simulink model "Multi_drones_deri_compare"  (R2021a)
settings: Solver=ode4  StartTime=0.0  StopTime=50  FixedStep=0.005  RelTol=1e-3
(part 1 of 7)
settings Model: Creator=a1752760  LastModifiedBy=a1752760

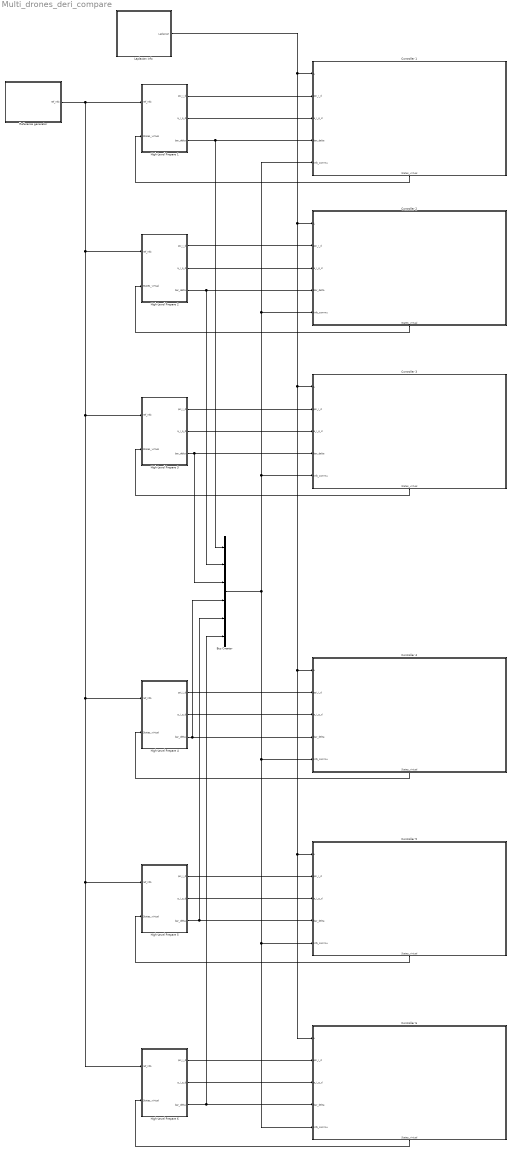
== system Multi_drones_deri_compare ==
  Bus Creator : BusCreator  Inputs=6
  Controller 1 : Subsystem
      settings: PortSchema="{\"entries\":[{\"content\":{\"sides\":[{\"content\":{\"connectorIds\":[\"In1\",\"In2\",\"In3\",\"In4\",\"In5\"]},\"type\":\"ConnectorPlacement.EquallySpacedRectSide\",\"uuid\":\"ede5c89e-e264-48e6-8668-eed849251501\"},{\"content\":{\"connectorIds\":[],\"side\":\"RIGHT\"},\"type\":\"ConnectorPlacement.EquallySpacedRectSide\",\"uuid\":\"e59691b4-d4b1-4407-a122-67eb4d4499aa\"},{\"content\":{\"connectorIds\":[],\"side\":\"TOP\"},\"type\":\"ConnectorPlacement.EquallySpacedRectSide\",\"uuid\":\"d9d52c18-65cc-4475-a64d-d3d1636b66e0\"},{\"content\":{\"connectorIds\":[\"Out1\"],\"side\":\"BOTTOM\"},\"type\":\"ConnectorPlacement.EquallySpacedRectSide\",\"uuid\":\"18635b8e-8039-4d54-8f78-9d501119f344\"}]},\"type\":\"ConnectorPlacement.EquallySpacedConnector\",\"uuid\":\"3cce6101-21cc-4dc7-9787-a7397180656f\"}],\"packageUris\":[\"http://schema.mathworks.com/mf0/Connector/R2020b\"],\"version\":\"1.0\"}"
  Controller 2 : Subsystem
      settings: PortSchema="{\"entries\":[{\"content\":{\"sides\":[{\"content\":{\"connectorIds\":[\"In1\",\"In2\",\"In3\",\"In4\",\"In5\"]},\"type\":\"ConnectorPlacement.EquallySpacedRectSide\",\"uuid\":\"ede5c89e-e264-48e6-8668-eed849251501\"},{\"content\":{\"connectorIds\":[],\"side\":\"RIGHT\"},\"type\":\"ConnectorPlacement.EquallySpacedRectSide\",\"uuid\":\"e59691b4-d4b1-4407-a122-67eb4d4499aa\"},{\"content\":{\"connectorIds\":[],\"side\":\"TOP\"},\"type\":\"ConnectorPlacement.EquallySpacedRectSide\",\"uuid\":\"d9d52c18-65cc-4475-a64d-d3d1636b66e0\"},{\"content\":{\"connectorIds\":[\"Out1\"],\"side\":\"BOTTOM\"},\"type\":\"ConnectorPlacement.EquallySpacedRectSide\",\"uuid\":\"18635b8e-8039-4d54-8f78-9d501119f344\"}]},\"type\":\"ConnectorPlacement.EquallySpacedConnector\",\"uuid\":\"3cce6101-21cc-4dc7-9787-a7397180656f\"}],\"packageUris\":[\"http://schema.mathworks.com/mf0/Connector/R2020b\"],\"version\":\"1.0\"}"
  Controller 3 : Subsystem
      settings: PortSchema="{\"entries\":[{\"content\":{\"sides\":[{\"content\":{\"connectorIds\":[\"In1\",\"In2\",\"In3\",\"In4\",\"In5\"]},\"type\":\"ConnectorPlacement.EquallySpacedRectSide\",\"uuid\":\"ede5c89e-e264-48e6-8668-eed849251501\"},{\"content\":{\"connectorIds\":[],\"side\":\"RIGHT\"},\"type\":\"ConnectorPlacement.EquallySpacedRectSide\",\"uuid\":\"e59691b4-d4b1-4407-a122-67eb4d4499aa\"},{\"content\":{\"connectorIds\":[],\"side\":\"TOP\"},\"type\":\"ConnectorPlacement.EquallySpacedRectSide\",\"uuid\":\"d9d52c18-65cc-4475-a64d-d3d1636b66e0\"},{\"content\":{\"connectorIds\":[\"Out1\"],\"side\":\"BOTTOM\"},\"type\":\"ConnectorPlacement.EquallySpacedRectSide\",\"uuid\":\"18635b8e-8039-4d54-8f78-9d501119f344\"}]},\"type\":\"ConnectorPlacement.EquallySpacedConnector\",\"uuid\":\"3cce6101-21cc-4dc7-9787-a7397180656f\"}],\"packageUris\":[\"http://schema.mathworks.com/mf0/Connector/R2020b\"],\"version\":\"1.0\"}"
  Controller 4 : Subsystem
      settings: PortSchema="{\"entries\":[{\"content\":{\"sides\":[{\"content\":{\"connectorIds\":[\"In1\",\"In2\",\"In3\",\"In4\",\"In5\"]},\"type\":\"ConnectorPlacement.EquallySpacedRectSide\",\"uuid\":\"ede5c89e-e264-48e6-8668-eed849251501\"},{\"content\":{\"connectorIds\":[],\"side\":\"RIGHT\"},\"type\":\"ConnectorPlacement.EquallySpacedRectSide\",\"uuid\":\"e59691b4-d4b1-4407-a122-67eb4d4499aa\"},{\"content\":{\"connectorIds\":[],\"side\":\"TOP\"},\"type\":\"ConnectorPlacement.EquallySpacedRectSide\",\"uuid\":\"d9d52c18-65cc-4475-a64d-d3d1636b66e0\"},{\"content\":{\"connectorIds\":[\"Out1\"],\"side\":\"BOTTOM\"},\"type\":\"ConnectorPlacement.EquallySpacedRectSide\",\"uuid\":\"18635b8e-8039-4d54-8f78-9d501119f344\"}]},\"type\":\"ConnectorPlacement.EquallySpacedConnector\",\"uuid\":\"3cce6101-21cc-4dc7-9787-a7397180656f\"}],\"packageUris\":[\"http://schema.mathworks.com/mf0/Connector/R2020b\"],\"version\":\"1.0\"}"
  Controller 5 : Subsystem
      settings: PortSchema="{\"entries\":[{\"content\":{\"sides\":[{\"content\":{\"connectorIds\":[\"In1\",\"In2\",\"In3\",\"In4\",\"In5\"]},\"type\":\"ConnectorPlacement.EquallySpacedRectSide\",\"uuid\":\"ede5c89e-e264-48e6-8668-eed849251501\"},{\"content\":{\"connectorIds\":[],\"side\":\"RIGHT\"},\"type\":\"ConnectorPlacement.EquallySpacedRectSide\",\"uuid\":\"e59691b4-d4b1-4407-a122-67eb4d4499aa\"},{\"content\":{\"connectorIds\":[],\"side\":\"TOP\"},\"type\":\"ConnectorPlacement.EquallySpacedRectSide\",\"uuid\":\"d9d52c18-65cc-4475-a64d-d3d1636b66e0\"},{\"content\":{\"connectorIds\":[\"Out1\"],\"side\":\"BOTTOM\"},\"type\":\"ConnectorPlacement.EquallySpacedRectSide\",\"uuid\":\"18635b8e-8039-4d54-8f78-9d501119f344\"}]},\"type\":\"ConnectorPlacement.EquallySpacedConnector\",\"uuid\":\"3cce6101-21cc-4dc7-9787-a7397180656f\"}],\"packageUris\":[\"http://schema.mathworks.com/mf0/Connector/R2020b\"],\"version\":\"1.0\"}"
  Controller 6 : Subsystem
      settings: PortSchema="{\"entries\":[{\"content\":{\"sides\":[{\"content\":{\"connectorIds\":[\"In1\",\"In2\",\"In3\",\"In4\",\"In5\"]},\"type\":\"ConnectorPlacement.EquallySpacedRectSide\",\"uuid\":\"ede5c89e-e264-48e6-8668-eed849251501\"},{\"content\":{\"connectorIds\":[],\"side\":\"RIGHT\"},\"type\":\"ConnectorPlacement.EquallySpacedRectSide\",\"uuid\":\"e59691b4-d4b1-4407-a122-67eb4d4499aa\"},{\"content\":{\"connectorIds\":[],\"side\":\"TOP\"},\"type\":\"ConnectorPlacement.EquallySpacedRectSide\",\"uuid\":\"d9d52c18-65cc-4475-a64d-d3d1636b66e0\"},{\"content\":{\"connectorIds\":[\"Out1\"],\"side\":\"BOTTOM\"},\"type\":\"ConnectorPlacement.EquallySpacedRectSide\",\"uuid\":\"18635b8e-8039-4d54-8f78-9d501119f344\"}]},\"type\":\"ConnectorPlacement.EquallySpacedConnector\",\"uuid\":\"3cce6101-21cc-4dc7-9787-a7397180656f\"}],\"packageUris\":[\"http://schema.mathworks.com/mf0/Connector/R2020b\"],\"version\":\"1.0\"}"
  High-Level Prepare 1 : Subsystem
  High-Level Prepare 2 : Subsystem
  High-Level Prepare 3 : Subsystem
  High-Level Prepare 4 : Subsystem
  High-Level Prepare 5 : Subsystem
  High-Level Prepare 6 : Subsystem
  Laplacian info : Subsystem
  Reference generator : Subsystem
  wires:
  Reference generator/1(ref_info) -> High-Level Prepare 6/1(ref_info), High-Level Prepare 5/1(ref_info), High-Level Prepare 4/1(ref_info), High-Level Prepare 3/1(ref_info), High-Level Prepare 2/1(ref_info), High-Level Prepare 1/1(ref_info)
  High-Level Prepare 1/1(psi_i_d) -> Controller 1/2(psi_i_d)
  High-Level Prepare 1/2(a_i_p_d) -> Controller 1/3(a_i_p_d)
  High-Level Prepare 1/3(bar_delta) -> Bus Creator/1, Controller 1/4(bar_delta)
  Controller 1/1(States_virtual) -> High-Level Prepare 1/2(States_virtual)
  Laplacian info/1(Laplacian) -> Controller 6/1(L), Controller 5/1(L), Controller 4/1(L), Controller 3/1(L), Controller 2/1(L), Controller 1/1(L)
  High-Level Prepare 2/2(a_i_p_d) -> Controller 2/3(a_i_p_d)
  High-Level Prepare 2/1(psi_i_d) -> Controller 2/2(psi_i_d)
  High-Level Prepare 2/3(bar_delta) -> Bus Creator/2, Controller 2/4(bar_delta)
  Controller 2/1(States_virtual) -> High-Level Prepare 2/2(States_virtual)
  High-Level Prepare 3/1(psi_i_d) -> Controller 3/2(psi_i_d)
  High-Level Prepare 3/3(bar_delta) -> Bus Creator/3, Controller 3/4(bar_delta)
  High-Level Prepare 3/2(a_i_p_d) -> Controller 3/3(a_i_p_d)
  Controller 3/1(States_virtual) -> High-Level Prepare 3/2(States_virtual)
  High-Level Prepare 4/1(psi_i_d) -> Controller 4/2(psi_i_d)
  High-Level Prepare 4/3(bar_delta) -> Bus Creator/4, Controller 4/4(bar_delta)
  High-Level Prepare 4/2(a_i_p_d) -> Controller 4/3(a_i_p_d)
  Controller 4/1(States_virtual) -> High-Level Prepare 4/2(States_virtual)
  High-Level Prepare 5/1(psi_i_d) -> Controller 5/2(psi_i_d)
  High-Level Prepare 5/3(bar_delta) -> Bus Creator/5, Controller 5/4(bar_delta)
  High-Level Prepare 5/2(a_i_p_d) -> Controller 5/3(a_i_p_d)
  Controller 5/1(States_virtual) -> High-Level Prepare 5/2(States_virtual)
  High-Level Prepare 6/1(psi_i_d) -> Controller 6/2(psi_i_d)
  High-Level Prepare 6/3(bar_delta) -> Bus Creator/6, Controller 6/4(bar_delta)
  High-Level Prepare 6/2(a_i_p_d) -> Controller 6/3(a_i_p_d)
  Controller 6/1(States_virtual) -> High-Level Prepare 6/2(States_virtual)
  Bus Creator/1 -> Controller 6/5(info_commu), Controller 5/5(info_commu), Controller 4/5(info_commu), Controller 2/5(info_commu), Controller 1/5(info_commu), Controller 3/5(info_commu)

== system Multi_drones_deri_compare/Controller 1 ==
  note: Change serial number and initial status
  note: Change serial number and initial status
  L : Inport
  psi_i_d : Inport  Port=2
  a_i_p_d : Inport  Port=3
  bar_delta : Inport  Port=4
  info_commu : Inport  Port=5
  Controller : Subsystem
  High-level system : Subsystem  mask{InitialCondition=[4;1;0]}
      mask prompts: InitialCondition "Simulink:blkprm_prompts:IntegratorInitCond"
      mask TypeOptions InitialCondition: bar_x/InitialCondition
      mask DialogControl InitialCondition Prompt: Initial condition:
  Quadcopter model : Subsystem  mask{InitialCondition=[4;1;0;0;0;0]}
      mask prompts: InitialCondition "Simulink:blkprm_prompts:IntegratorInitCond"
      mask TypeOptions InitialCondition: x_int/InitialCondition
      mask DialogControl InitialCondition Prompt: Initial condition:
  States_virtual : Outport
  wires:
  info_commu/1 -> High-level system/2(info_commu)
  bar_delta/1 -> High-level system/3(bar_delta)
  L/1 -> High-level system/1(L)
  a_i_p_d/1 -> High-level system/4(a_d)
  High-level system/2(States_virtual) -> States_virtual/1
  Controller/2(w_hat_p) -> Quadcopter model/2(w_hat_p)
  Quadcopter model/1(states_i) -> Controller/1(states_i)
  Controller/1(u_i) -> Quadcopter model/1(u_i)
  Controller/3(w_hat_a) -> Quadcopter model/3(w_hat_a)
  psi_i_d/1 -> Controller/3(psi_id)
  High-level system/1(new_ref) -> Controller/2(ref_x_p)

== system Multi_drones_deri_compare/Controller 2 ==
  note: Change serial number and initial status
  note: Change serial number and initial status
  L : Inport
  psi_i_d : Inport  Port=2
  a_i_p_d : Inport  Port=3
  bar_delta : Inport  Port=4
  info_commu : Inport  Port=5
  Controller : Subsystem
  High-level system : Subsystem  mask{InitialCondition=[1;2;0]}
      mask prompts: InitialCondition "Simulink:blkprm_prompts:IntegratorInitCond"
      mask TypeOptions InitialCondition: bar_x/InitialCondition
      mask DialogControl InitialCondition Prompt: Initial condition:
  Quadcopter model : Subsystem  mask{InitialCondition=[1;2;0;0;0;0]}
      mask prompts: InitialCondition "Simulink:blkprm_prompts:IntegratorInitCond"
      mask TypeOptions InitialCondition: x_int/InitialCondition
      mask DialogControl InitialCondition Prompt: Initial condition:
  States_virtual : Outport
  wires:
  info_commu/1 -> High-level system/2(info_commu)
  bar_delta/1 -> High-level system/3(bar_delta)
  L/1 -> High-level system/1(L)
  a_i_p_d/1 -> High-level system/4(a_d)
  High-level system/2(States_virtual) -> States_virtual/1
  Controller/2(w_hat_p) -> Quadcopter model/2(w_hat_p)
  Quadcopter model/1(states_i) -> Controller/1(states_i)
  Controller/1(u_i) -> Quadcopter model/1(u_i)
  Controller/3(w_hat_a) -> Quadcopter model/3(w_hat_a)
  psi_i_d/1 -> Controller/3(psi_id)
  High-level system/1(new_ref) -> Controller/2(ref_x_p)

== system Multi_drones_deri_compare/Controller 3 ==
  note: Change serial number and initial status
  note: Change serial number and initial status
  L : Inport
  psi_i_d : Inport  Port=2
  a_i_p_d : Inport  Port=3
  bar_delta : Inport  Port=4
  info_commu : Inport  Port=5
  Controller : Subsystem
  High-level system : Subsystem  mask{InitialCondition=[-2;4;0]}
      mask prompts: InitialCondition "Simulink:blkprm_prompts:IntegratorInitCond"
      mask TypeOptions InitialCondition: bar_x/InitialCondition
      mask DialogControl InitialCondition Prompt: Initial condition:
  Quadcopter model : Subsystem  mask{InitialCondition=[-2;4;0;0;0;0]}
      mask prompts: InitialCondition "Simulink:blkprm_prompts:IntegratorInitCond"
      mask TypeOptions InitialCondition: x_int/InitialCondition
      mask DialogControl InitialCondition Prompt: Initial condition:
  States_virtual : Outport
  wires:
  info_commu/1 -> High-level system/2(info_commu)
  bar_delta/1 -> High-level system/3(bar_delta)
  L/1 -> High-level system/1(L)
  a_i_p_d/1 -> High-level system/4(a_d)
  High-level system/2(States_virtual) -> States_virtual/1
  Controller/2(w_hat_p) -> Quadcopter model/2(w_hat_p)
  Quadcopter model/1(states_i) -> Controller/1(states_i)
  Controller/1(u_i) -> Quadcopter model/1(u_i)
  Controller/3(w_hat_a) -> Quadcopter model/3(w_hat_a)
  psi_i_d/1 -> Controller/3(psi_id)
  High-level system/1(new_ref) -> Controller/2(ref_x_p)

== system Multi_drones_deri_compare/Controller 4 ==
  note: Change serial number and initial status
  note: Change serial number and initial status
  L : Inport
  psi_i_d : Inport  Port=2
  a_i_p_d : Inport  Port=3
  bar_delta : Inport  Port=4
  info_commu : Inport  Port=5
  Controller : Subsystem
  High-level system : Subsystem  mask{InitialCondition=[-4;-1;0]}
      mask prompts: InitialCondition "Simulink:blkprm_prompts:IntegratorInitCond"
      mask TypeOptions InitialCondition: bar_x/InitialCondition
      mask DialogControl InitialCondition Prompt: Initial condition:
  Quadcopter model : Subsystem  mask{InitialCondition=[-4;-1;0;0;0;0]}
      mask prompts: InitialCondition "Simulink:blkprm_prompts:IntegratorInitCond"
      mask TypeOptions InitialCondition: x_int/InitialCondition
      mask DialogControl InitialCondition Prompt: Initial condition:
  States_virtual : Outport
  wires:
  info_commu/1 -> High-level system/2(info_commu)
  bar_delta/1 -> High-level system/3(bar_delta)
  L/1 -> High-level system/1(L)
  a_i_p_d/1 -> High-level system/4(a_d)
  High-level system/2(States_virtual) -> States_virtual/1
  Controller/2(w_hat_p) -> Quadcopter model/2(w_hat_p)
  Quadcopter model/1(states_i) -> Controller/1(states_i)
  Controller/1(u_i) -> Quadcopter model/1(u_i)
  Controller/3(w_hat_a) -> Quadcopter model/3(w_hat_a)
  psi_i_d/1 -> Controller/3(psi_id)
  High-level system/1(new_ref) -> Controller/2(ref_x_p)

== system Multi_drones_deri_compare/Controller 5 ==
  note: Change serial number and initial status
  note: Change serial number and initial status
  L : Inport
  psi_i_d : Inport  Port=2
  a_i_p_d : Inport  Port=3
  bar_delta : Inport  Port=4
  info_commu : Inport  Port=5
  Controller : Subsystem
  High-level system : Subsystem  mask{InitialCondition=[-1.5;-1;0]}
      mask prompts: InitialCondition "Simulink:blkprm_prompts:IntegratorInitCond"
      mask TypeOptions InitialCondition: bar_x/InitialCondition
      mask DialogControl InitialCondition Prompt: Initial condition:
  Quadcopter model : Subsystem  mask{InitialCondition=[-1.5;-1;0;0;0;0]}
      mask prompts: InitialCondition "Simulink:blkprm_prompts:IntegratorInitCond"
      mask TypeOptions InitialCondition: x_int/InitialCondition
      mask DialogControl InitialCondition Prompt: Initial condition:
  States_virtual : Outport
  wires:
  info_commu/1 -> High-level system/2(info_commu)
  bar_delta/1 -> High-level system/3(bar_delta)
  L/1 -> High-level system/1(L)
  a_i_p_d/1 -> High-level system/4(a_d)
  High-level system/2(States_virtual) -> States_virtual/1
  Controller/2(w_hat_p) -> Quadcopter model/2(w_hat_p)
  Quadcopter model/1(states_i) -> Controller/1(states_i)
  Controller/1(u_i) -> Quadcopter model/1(u_i)
  Controller/3(w_hat_a) -> Quadcopter model/3(w_hat_a)
  psi_i_d/1 -> Controller/3(psi_id)
  High-level system/1(new_ref) -> Controller/2(ref_x_p)

== system Multi_drones_deri_compare/Controller 6 ==
  note: Change serial number and initial status
  note: Change serial number and initial status
  L : Inport
  psi_i_d : Inport  Port=2
  a_i_p_d : Inport  Port=3
  bar_delta : Inport  Port=4
  info_commu : Inport  Port=5
  Controller : Subsystem
  High-level system : Subsystem  mask{InitialCondition=[0;-1;0]}
      mask prompts: InitialCondition "Simulink:blkprm_prompts:IntegratorInitCond"
      mask TypeOptions InitialCondition: bar_x/InitialCondition
      mask DialogControl InitialCondition Prompt: Initial condition:
  Quadcopter model : Subsystem  mask{InitialCondition=[0;-1;0;0;0;0]}
      mask prompts: InitialCondition "Simulink:blkprm_prompts:IntegratorInitCond"
      mask TypeOptions InitialCondition: x_int/InitialCondition
      mask DialogControl InitialCondition Prompt: Initial condition:
  States_virtual : Outport
  wires:
  info_commu/1 -> High-level system/2(info_commu)
  bar_delta/1 -> High-level system/3(bar_delta)
  L/1 -> High-level system/1(L)
  a_i_p_d/1 -> High-level system/4(a_d)
  High-level system/2(States_virtual) -> States_virtual/1
  Controller/2(w_hat_p) -> Quadcopter model/2(w_hat_p)
  Quadcopter model/1(states_i) -> Controller/1(states_i)
  Controller/1(u_i) -> Quadcopter model/1(u_i)
  Controller/3(w_hat_a) -> Quadcopter model/3(w_hat_a)
  psi_i_d/1 -> Controller/3(psi_id)
  High-level system/1(new_ref) -> Controller/2(ref_x_p)

== system Multi_drones_deri_compare/High-Level Prepare 1 ==
  note: Change serial number here
  ref_info : Inport
  States_virtual : Inport  Port=2
  Bus Creator : BusCreator  Inputs=2
  Reference selection (Low) : MATLAB Function  TreatAsAtomicUnit=on
  States selection (Virtual) : MATLAB Function  TreatAsAtomicUnit=on
  Virtual error calculation : MATLAB Function  TreatAsAtomicUnit=on
  psi_i_d : Outport
  a_i_p_d : Outport  Port=2
  bar_delta : Outport  Port=3
  wires:
  ref_info/1 -> Reference selection (Low)/1(ref_info)
  Reference selection (Low)/4(psi_i_d) -> psi_i_d/1
  States_virtual/1 -> States selection (Virtual)/1(states_virtual)
  Reference selection (Low)/3(a_i_p_d) -> a_i_p_d/1
  States selection (Virtual)/2(v_bar_i) -> Virtual error calculation/2(v_bar_i)
  States selection (Virtual)/1(x_bar_i) -> Virtual error calculation/1(x_bar_i)
  Reference selection (Low)/1(x_i_p_d) -> Virtual error calculation/3(x_i_p_d)
  Reference selection (Low)/2(v_i_p_d) -> Virtual error calculation/4(v_i_p_d)
  Virtual error calculation/1(bar_delta_x) -> Bus Creator/1
  Virtual error calculation/2(bar_delta_v) -> Bus Creator/2
  Bus Creator/1 -> bar_delta/1

== system Multi_drones_deri_compare/High-Level Prepare 2 ==
  note: Change serial number here
  ref_info : Inport
  States_virtual : Inport  Port=2
  Bus Creator : BusCreator  Inputs=2
  Reference selection (Low) : MATLAB Function  TreatAsAtomicUnit=on
  States selection (Virtual) : MATLAB Function  TreatAsAtomicUnit=on
  Virtual error calculation : MATLAB Function  TreatAsAtomicUnit=on
  psi_i_d : Outport
  a_i_p_d : Outport  Port=2
  bar_delta : Outport  Port=3
  wires:
  ref_info/1 -> Reference selection (Low)/1(ref_info)
  Reference selection (Low)/4(psi_i_d) -> psi_i_d/1
  States_virtual/1 -> States selection (Virtual)/1(states_virtual)
  Reference selection (Low)/3(a_i_p_d) -> a_i_p_d/1
  States selection (Virtual)/2(v_bar_i) -> Virtual error calculation/2(v_bar_i)
  States selection (Virtual)/1(x_bar_i) -> Virtual error calculation/1(x_bar_i)
  Reference selection (Low)/1(x_i_p_d) -> Virtual error calculation/3(x_i_p_d)
  Reference selection (Low)/2(v_i_p_d) -> Virtual error calculation/4(v_i_p_d)
  Virtual error calculation/1(bar_delta_x) -> Bus Creator/1
  Virtual error calculation/2(bar_delta_v) -> Bus Creator/2
  Bus Creator/1 -> bar_delta/1

== system Multi_drones_deri_compare/High-Level Prepare 3 ==
  note: Change serial number here
  ref_info : Inport
  States_virtual : Inport  Port=2
  Bus Creator : BusCreator  Inputs=2
  Reference selection (Low) : MATLAB Function  TreatAsAtomicUnit=on
  States selection (Virtual) : MATLAB Function  TreatAsAtomicUnit=on
  Virtual error calculation : MATLAB Function  TreatAsAtomicUnit=on
  psi_i_d : Outport
  a_i_p_d : Outport  Port=2
  bar_delta : Outport  Port=3
  wires:
  ref_info/1 -> Reference selection (Low)/1(ref_info)
  Reference selection (Low)/4(psi_i_d) -> psi_i_d/1
  States_virtual/1 -> States selection (Virtual)/1(states_virtual)
  Reference selection (Low)/3(a_i_p_d) -> a_i_p_d/1
  States selection (Virtual)/2(v_bar_i) -> Virtual error calculation/2(v_bar_i)
  States selection (Virtual)/1(x_bar_i) -> Virtual error calculation/1(x_bar_i)
  Reference selection (Low)/1(x_i_p_d) -> Virtual error calculation/3(x_i_p_d)
  Reference selection (Low)/2(v_i_p_d) -> Virtual error calculation/4(v_i_p_d)
  Virtual error calculation/1(bar_delta_x) -> Bus Creator/1
  Virtual error calculation/2(bar_delta_v) -> Bus Creator/2
  Bus Creator/1 -> bar_delta/1

== system Multi_drones_deri_compare/High-Level Prepare 4 ==
  note: Change serial number here
  ref_info : Inport
  States_virtual : Inport  Port=2
  Bus Creator : BusCreator  Inputs=2
  Reference selection (Low) : MATLAB Function  TreatAsAtomicUnit=on
  States selection (Virtual) : MATLAB Function  TreatAsAtomicUnit=on
  Virtual error calculation : MATLAB Function  TreatAsAtomicUnit=on
  psi_i_d : Outport
  a_i_p_d : Outport  Port=2
  bar_delta : Outport  Port=3
  wires:
  ref_info/1 -> Reference selection (Low)/1(ref_info)
  Reference selection (Low)/4(psi_i_d) -> psi_i_d/1
  States_virtual/1 -> States selection (Virtual)/1(states_virtual)
  Reference selection (Low)/3(a_i_p_d) -> a_i_p_d/1
  States selection (Virtual)/2(v_bar_i) -> Virtual error calculation/2(v_bar_i)
  States selection (Virtual)/1(x_bar_i) -> Virtual error calculation/1(x_bar_i)
  Reference selection (Low)/1(x_i_p_d) -> Virtual error calculation/3(x_i_p_d)
  Reference selection (Low)/2(v_i_p_d) -> Virtual error calculation/4(v_i_p_d)
  Virtual error calculation/1(bar_delta_x) -> Bus Creator/1
  Virtual error calculation/2(bar_delta_v) -> Bus Creator/2
  Bus Creator/1 -> bar_delta/1

== system Multi_drones_deri_compare/High-Level Prepare 5 ==
  note: Change serial number here
  ref_info : Inport
  States_virtual : Inport  Port=2
  Bus Creator : BusCreator  Inputs=2
  Reference selection (Low) : MATLAB Function  TreatAsAtomicUnit=on
  States selection (Virtual) : MATLAB Function  TreatAsAtomicUnit=on
  Virtual error calculation : MATLAB Function  TreatAsAtomicUnit=on
  psi_i_d : Outport
  a_i_p_d : Outport  Port=2
  bar_delta : Outport  Port=3
  wires:
  ref_info/1 -> Reference selection (Low)/1(ref_info)
  Reference selection (Low)/4(psi_i_d) -> psi_i_d/1
  States_virtual/1 -> States selection (Virtual)/1(states_virtual)
  Reference selection (Low)/3(a_i_p_d) -> a_i_p_d/1
  States selection (Virtual)/2(v_bar_i) -> Virtual error calculation/2(v_bar_i)
  States selection (Virtual)/1(x_bar_i) -> Virtual error calculation/1(x_bar_i)
  Reference selection (Low)/1(x_i_p_d) -> Virtual error calculation/3(x_i_p_d)
  Reference selection (Low)/2(v_i_p_d) -> Virtual error calculation/4(v_i_p_d)
  Virtual error calculation/1(bar_delta_x) -> Bus Creator/1
  Virtual error calculation/2(bar_delta_v) -> Bus Creator/2
  Bus Creator/1 -> bar_delta/1

== system Multi_drones_deri_compare/High-Level Prepare 6 ==
  note: Change serial number here
  ref_info : Inport
  States_virtual : Inport  Port=2
  Bus Creator : BusCreator  Inputs=2
  Reference selection (Low) : MATLAB Function  TreatAsAtomicUnit=on
  States selection (Virtual) : MATLAB Function  TreatAsAtomicUnit=on
  Virtual error calculation : MATLAB Function  TreatAsAtomicUnit=on
  psi_i_d : Outport
  a_i_p_d : Outport  Port=2
  bar_delta : Outport  Port=3
  wires:
  ref_info/1 -> Reference selection (Low)/1(ref_info)
  Reference selection (Low)/4(psi_i_d) -> psi_i_d/1
  States_virtual/1 -> States selection (Virtual)/1(states_virtual)
  Reference selection (Low)/3(a_i_p_d) -> a_i_p_d/1
  States selection (Virtual)/2(v_bar_i) -> Virtual error calculation/2(v_bar_i)
  States selection (Virtual)/1(x_bar_i) -> Virtual error calculation/1(x_bar_i)
  Reference selection (Low)/1(x_i_p_d) -> Virtual error calculation/3(x_i_p_d)
  Reference selection (Low)/2(v_i_p_d) -> Virtual error calculation/4(v_i_p_d)
  Virtual error calculation/1(bar_delta_x) -> Bus Creator/1
  Virtual error calculation/2(bar_delta_v) -> Bus Creator/2
  Bus Creator/1 -> bar_delta/1

== system Multi_drones_deri_compare/Laplacian info ==
  Add : Sum
  Communication topology : MATLAB Function  TreatAsAtomicUnit=on
  Constant : Constant  Value=diag(ones(6,1))  VectorParams1D=off
  Multiply : Gain
  Laplacian : Outport
  wires:
  Constant/1 -> Multiply/1
  Multiply/1 -> Add/1
  Add/1 -> Laplacian/1
  Communication topology/1(L) -> Add/2

== system Multi_drones_deri_compare/Reference generator ==
  Bus Creator : BusCreator  Inputs=4
  Coordinate reference : Subsystem
  MATLAB Function : MATLAB Function  TreatAsAtomicUnit=on
  Scope : Scope
  Simulation time : Clock
  ref_info : Outport
  wires:
  Simulation time/1 -> Coordinate reference/1(Time), MATLAB Function/1(t)
  Coordinate reference/1(x_d_p) -> Scope/1, Bus Creator/1
  Coordinate reference/2(v_d_p) -> Bus Creator/2
  Coordinate reference/3(a_d_p) -> Bus Creator/3
  MATLAB Function/1(x_d_a) -> Bus Creator/4
  Bus Creator/1 -> ref_info/1

== system Multi_drones_deri_compare/Controller 1/Controller ==
  note: Change the serial number here
  note: Change the serial number here
  note: Change the serial number here
  states_i : Inport
  ref_x_p : Inport  Port=2
  psi_id : Inport  Port=3
  Attitude controller : Subsystem
      settings: PortSchema="{\"entries\":[{\"content\":{\"sides\":[{\"content\":{\"connectorIds\":[\"In1\",\"In2\",\"In3\"]},\"type\":\"ConnectorPlacement.EquallySpacedRectSide\",\"uuid\":\"fa62b1eb-ed3d-4a84-b897-b51f17bb9d42\"},{\"content\":{\"connectorIds\":[\"Out1\"],\"side\":\"RIGHT\"},\"type\":\"ConnectorPlacement.EquallySpacedRectSide\",\"uuid\":\"9b6b7a3c-e484-45bf-bd32-fe40ffeb0d28\"},{\"content\":{\"connectorIds\":[\"Out2\"],\"side\":\"TOP\"},\"type\":\"ConnectorPlacement.EquallySpacedRectSide\",\"uuid\":\"d1ffdbb9-18c9-4f2c-95a6-bf4c2ab27347\"}]},\"type\":\"ConnectorPlacement.EquallySpacedConnector\",\"uuid\":\"2804a1df-60db-43d6-95d2-4687dde4bd06\"}],\"packageUris\":[\"http://schema.mathworks.com/mf0/Connector/R2020b\"],\"version\":\"1.0\"}"
  Constant : Constant  Value=13.72  VectorParams1D=off
  Manual Switch : ManualSwitch
  Nominal control calculation : MATLAB Function  TreatAsAtomicUnit=on
  Position controller1 : Subsystem
      settings: PortSchema="{\"entries\":[{\"content\":{\"sides\":[{\"content\":{\"connectorIds\":[\"In1\",\"In2\",\"In3\"]},\"type\":\"ConnectorPlacement.EquallySpacedRectSide\",\"uuid\":\"6f6db54a-065c-4c68-96d3-ce6f9528f7c2\"},{\"content\":{\"connectorIds\":[\"Out1\"],\"side\":\"RIGHT\"},\"type\":\"ConnectorPlacement.EquallySpacedRectSide\",\"uuid\":\"eab021de-0481-49e0-8239-dbc5993eb5fa\"},{\"content\":{\"connectorIds\":[\"Out2\"],\"side\":\"TOP\"},\"type\":\"ConnectorPlacement.EquallySpacedRectSide\",\"uuid\":\"c7d044cf-1b8b-40e5-8601-940ebebd0ccb\"},{\"content\":{\"connectorIds\":[],\"side\":\"BOTTOM\"},\"type\":\"ConnectorPlacement.EquallySpacedRectSide\",\"uuid\":\"6c5daa93-b438-4c34-9741-3ab1f6346320\"}]},\"type\":\"ConnectorPlacement.EquallySpacedConnector\",\"uuid\":\"bb7db914-9823-41d6-a8ba-39b4d2976335\"}],\"packageUris\":[\"http://schema.mathworks.com/mf0/Connector/R2020b\"],\"version\":\"1.0\"}"
  Real control input : MATLAB Function  TreatAsAtomicUnit=on
  Reverse calculation : Subsystem
      settings: PortSchema="{\"entries\":[{\"content\":{\"sides\":[{\"content\":{\"connectorIds\":[\"In1\",\"In2\"]},\"type\":\"ConnectorPlacement.EquallySpacedRectSide\",\"uuid\":\"a324fb00-881d-40c1-b7da-a9c7871d46ce\"},{\"content\":{\"connectorIds\":[\"Out1\",\"Out2\"],\"side\":\"RIGHT\"},\"type\":\"ConnectorPlacement.EquallySpacedRectSide\",\"uuid\":\"58739d0b-b2b3-44e8-8796-6553ce8d5a15\"},{\"content\":{\"connectorIds\":[\"In3\"],\"side\":\"TOP\"},\"type\":\"ConnectorPlacement.EquallySpacedRectSide\",\"uuid\":\"8c9acd48-a842-4889-b739-8799f04ac800\"}]},\"type\":\"ConnectorPlacement.EquallySpacedConnector\",\"uuid\":\"9c847f57-6425-42e5-8be7-b64809e08636\"}],\"packageUris\":[\"http://schema.mathworks.com/mf0/Connector/R2020b\"],\"version\":\"1.0\"}"
  Scope : Scope
  T_id : Scope
  atti_ref : Scope
  u : Scope
  u_ip : Scope
  u_nom_a : Scope
  u_nom_p : Scope
  u_i : Outport
  w_hat_p : Outport  Port=2
  w_hat_a : Outport  Port=3
  wires:
  Attitude controller/1(u_I_a) -> Real control input/1(u_i_a)
  ref_x_p/1 -> Position controller1/2(ref_x_p)
  states_i/1 -> Position controller1/1(states_i), Reverse calculation/3(states_i), Attitude controller/1(states_i), Nominal control calculation/1(states_i)
  Nominal control calculation/1(u_nom_p) -> Position controller1/3(u_nom_p), u_nom_p/1
  Nominal control calculation/2(u_nom_a) -> Attitude controller/3(u_nom_a), u_nom_a/1
  Position controller1/1(u_i_p) -> Reverse calculation/2(u_ip), u_ip/1
  Reverse calculation/1(atti_ref) -> Attitude controller/2(atti_ref), atti_ref/1
  Position controller1/2(w_hat_p) -> w_hat_p/1
  Attitude controller/2(w_hat_a) -> w_hat_a/1
  Constant/1 -> Manual Switch/2
  Reverse calculation/2(T_i_d) -> Manual Switch/1
  Manual Switch/1 -> T_id/1, Real control input/2(T_id)
  Real control input/2(u_i) -> Nominal control calculation/2(u_i), u/1, u_i/1
  Real control input/1(tau_i) -> Scope/1
  psi_id/1 -> Reverse calculation/1(psi_id)

== system Multi_drones_deri_compare/Controller 1/High-level system ==
  L : Inport
  info_commu : Inport  Port=2
  bar_delta : Inport  Port=3
  a_d : Inport  Port=4
  Bus Creator : BusCreator  Inputs=3
  Bus Creator1 : BusCreator  Inputs=2
  Controller : MATLAB Function  TreatAsAtomicUnit=on
  Information subtracting : MATLAB Function  TreatAsAtomicUnit=on
  Saturation : Saturate  UpperLimit=0.2  LowerLimit=-0.2
  Virtual sliding variable : Scope
  Virtual tracking error : Scope
  bar_u_i : Scope
  bar_v : Integrator  InitialCondition=[0;0;0]  ContinuousStateAttributes='speed'
  bar_v_i : Scope
  bar_x : Integrator  Tag=Position_x1  InitialCondition=InitialCondition  ContinuousStateAttributes='position'
  bar_x_i : Scope
  new_ref : Outport
  States_virtual : Outport  Port=2
  wires:
  Information subtracting/1(delta_xi) -> Controller/1(delta_xi), Virtual tracking error/1
  Information subtracting/2(delta_vi) -> Controller/2(delta_vi)
  Information subtracting/3(s_i) -> Virtual sliding variable/1, Controller/3(s_i)
  info_commu/1 -> Information subtracting/2(info_commu)
  bar_delta/1 -> Information subtracting/3(bar_delta)
  L/1 -> Information subtracting/1(L)
  a_d/1 -> Controller/5(a_di)
  bar_v/1 -> Bus Creator1/2, bar_v_i/1, Bus Creator/2, bar_x/1
  Bus Creator/1 -> new_ref/1
  bar_x/1 -> Bus Creator1/1, Bus Creator/1, bar_x_i/1
  Bus Creator1/1 -> States_virtual/1
  Controller/1(u_i) -> Saturation/1
  Saturation/1 -> bar_u_i/1, Bus Creator/3, bar_v/1
  Information subtracting/4(sat_dot) -> Controller/4(sat_dot)

== system Multi_drones_deri_compare/Controller 1/Quadcopter model ==
  u_i : Inport
  w_hat_p : Inport  Port=2
  w_hat_a : Inport  Port=3
  Add : Sum  Inputs=+-
  Add1 : Sum  Inputs=+-
  Bus Creator : BusCreator  Inputs=2
  Clock : Clock
  Quadcopter dynamics : MATLAB Function  TreatAsAtomicUnit=on
  f_a : Scope
  f_p : Scope
  quad_v : Scope
  quad_x : Scope
  v_int : Integrator  InitialCondition=[0;0;0;0;0;0]
  w_tilde_a : Scope
  w_tilde_p : Scope
  x_int : Integrator  InitialCondition=InitialCondition
  states_i : Outport
  wires:
  u_i/1 -> Quadcopter dynamics/2(u_i)
  Quadcopter dynamics/1(x_ddot) -> v_int/1
  x_int/1 -> Quadcopter dynamics/1(x_i), quad_x/1, Bus Creator/1
  v_int/1 -> Bus Creator/2, quad_v/1, Quadcopter dynamics/4(v_i), x_int/1
  Bus Creator/1 -> states_i/1
  Quadcopter dynamics/2(w_a) -> Add/1, f_a/1
  w_hat_a/1 -> Add/2
  Add/1 -> w_tilde_a/1
  Clock/1 -> Quadcopter dynamics/3(t)
  Quadcopter dynamics/3(w_p) -> f_p/1, Add1/1
  w_hat_p/1 -> Add1/2
  Add1/1 -> w_tilde_p/1

== system Multi_drones_deri_compare/Controller 2/Controller ==
  note: Change the serial number here
  note: Change the serial number here
  note: Change the serial number here
  states_i : Inport
  ref_x_p : Inport  Port=2
  psi_id : Inport  Port=3
  Attitude controller : Subsystem
      settings: PortSchema="{\"entries\":[{\"content\":{\"sides\":[{\"content\":{\"connectorIds\":[\"In1\",\"In2\",\"In3\"]},\"type\":\"ConnectorPlacement.EquallySpacedRectSide\",\"uuid\":\"fa62b1eb-ed3d-4a84-b897-b51f17bb9d42\"},{\"content\":{\"connectorIds\":[\"Out1\"],\"side\":\"RIGHT\"},\"type\":\"ConnectorPlacement.EquallySpacedRectSide\",\"uuid\":\"9b6b7a3c-e484-45bf-bd32-fe40ffeb0d28\"},{\"content\":{\"connectorIds\":[\"Out2\"],\"side\":\"TOP\"},\"type\":\"ConnectorPlacement.EquallySpacedRectSide\",\"uuid\":\"d1ffdbb9-18c9-4f2c-95a6-bf4c2ab27347\"}]},\"type\":\"ConnectorPlacement.EquallySpacedConnector\",\"uuid\":\"2804a1df-60db-43d6-95d2-4687dde4bd06\"}],\"packageUris\":[\"http://schema.mathworks.com/mf0/Connector/R2020b\"],\"version\":\"1.0\"}"
  Constant : Constant  Value=13.72  VectorParams1D=off
  Manual Switch : ManualSwitch
  Nominal control calculation : MATLAB Function  TreatAsAtomicUnit=on
  Position controller1 : Subsystem
      settings: PortSchema="{\"entries\":[{\"content\":{\"sides\":[{\"content\":{\"connectorIds\":[\"In1\",\"In2\",\"In3\"]},\"type\":\"ConnectorPlacement.EquallySpacedRectSide\",\"uuid\":\"6f6db54a-065c-4c68-96d3-ce6f9528f7c2\"},{\"content\":{\"connectorIds\":[\"Out1\"],\"side\":\"RIGHT\"},\"type\":\"ConnectorPlacement.EquallySpacedRectSide\",\"uuid\":\"eab021de-0481-49e0-8239-dbc5993eb5fa\"},{\"content\":{\"connectorIds\":[\"Out2\"],\"side\":\"TOP\"},\"type\":\"ConnectorPlacement.EquallySpacedRectSide\",\"uuid\":\"c7d044cf-1b8b-40e5-8601-940ebebd0ccb\"},{\"content\":{\"connectorIds\":[],\"side\":\"BOTTOM\"},\"type\":\"ConnectorPlacement.EquallySpacedRectSide\",\"uuid\":\"6c5daa93-b438-4c34-9741-3ab1f6346320\"}]},\"type\":\"ConnectorPlacement.EquallySpacedConnector\",\"uuid\":\"bb7db914-9823-41d6-a8ba-39b4d2976335\"}],\"packageUris\":[\"http://schema.mathworks.com/mf0/Connector/R2020b\"],\"version\":\"1.0\"}"
  Real control input : MATLAB Function  TreatAsAtomicUnit=on
  Reverse calculation : Subsystem
      settings: PortSchema="{\"entries\":[{\"content\":{\"sides\":[{\"content\":{\"connectorIds\":[\"In1\",\"In2\"]},\"type\":\"ConnectorPlacement.EquallySpacedRectSide\",\"uuid\":\"a324fb00-881d-40c1-b7da-a9c7871d46ce\"},{\"content\":{\"connectorIds\":[\"Out1\",\"Out2\"],\"side\":\"RIGHT\"},\"type\":\"ConnectorPlacement.EquallySpacedRectSide\",\"uuid\":\"58739d0b-b2b3-44e8-8796-6553ce8d5a15\"},{\"content\":{\"connectorIds\":[\"In3\"],\"side\":\"TOP\"},\"type\":\"ConnectorPlacement.EquallySpacedRectSide\",\"uuid\":\"8c9acd48-a842-4889-b739-8799f04ac800\"}]},\"type\":\"ConnectorPlacement.EquallySpacedConnector\",\"uuid\":\"9c847f57-6425-42e5-8be7-b64809e08636\"}],\"packageUris\":[\"http://schema.mathworks.com/mf0/Connector/R2020b\"],\"version\":\"1.0\"}"
  Scope : Scope
  T_id : Scope
  atti_ref : Scope
  u : Scope
  u_ip : Scope
  u_nom_a : Scope
  u_nom_p : Scope
  u_i : Outport
  w_hat_p : Outport  Port=2
  w_hat_a : Outport  Port=3
  wires:
  Attitude controller/1(u_I_a) -> Real control input/1(u_i_a)
  ref_x_p/1 -> Position controller1/2(ref_x_p)
  states_i/1 -> Position controller1/1(states_i), Reverse calculation/3(states_i), Attitude controller/1(states_i), Nominal control calculation/1(states_i)
  Nominal control calculation/1(u_nom_p) -> Position controller1/3(u_nom_p), u_nom_p/1
  Nominal control calculation/2(u_nom_a) -> Attitude controller/3(u_nom_a), u_nom_a/1
  Position controller1/1(u_i_p) -> Reverse calculation/2(u_ip), u_ip/1
  Reverse calculation/1(atti_ref) -> Attitude controller/2(atti_ref), atti_ref/1
  Position controller1/2(w_hat_p) -> w_hat_p/1
  Attitude controller/2(w_hat_a) -> w_hat_a/1
  Constant/1 -> Manual Switch/2
  Reverse calculation/2(T_i_d) -> Manual Switch/1
  Manual Switch/1 -> T_id/1, Real control input/2(T_id)
  Real control input/2(u_i) -> Nominal control calculation/2(u_i), u/1, u_i/1
  Real control input/1(tau_i) -> Scope/1
  psi_id/1 -> Reverse calculation/1(psi_id)

== system Multi_drones_deri_compare/Controller 2/High-level system ==
  L : Inport
  info_commu : Inport  Port=2
  bar_delta : Inport  Port=3
  a_d : Inport  Port=4
  Bus Creator : BusCreator  Inputs=3
  Bus Creator1 : BusCreator  Inputs=2
  Controller : MATLAB Function  TreatAsAtomicUnit=on
  Information subtracting : MATLAB Function  TreatAsAtomicUnit=on
  Saturation : Saturate  UpperLimit=0.2  LowerLimit=-0.2
  Virtual sliding variable : Scope
  Virtual tracking error : Scope
  bar_u_i : Scope
  bar_v : Integrator  InitialCondition=[0;0;0]  ContinuousStateAttributes='speed'
  bar_v_i : Scope
  bar_x : Integrator  Tag=Position_x1  InitialCondition=InitialCondition  ContinuousStateAttributes='position'
  bar_x_i : Scope
  new_ref : Outport
  States_virtual : Outport  Port=2
  wires:
  Information subtracting/1(delta_xi) -> Controller/1(delta_xi), Virtual tracking error/1
  Information subtracting/4(sat_dot) -> Controller/4(sat_dot)
  info_commu/1 -> Information subtracting/2(info_commu)
  bar_delta/1 -> Information subtracting/3(bar_delta)
  L/1 -> Information subtracting/1(L)
  a_d/1 -> Controller/5(a_di)
  bar_v/1 -> Bus Creator1/2, bar_v_i/1, Bus Creator/2, bar_x/1
  Bus Creator/1 -> new_ref/1
  bar_x/1 -> Bus Creator1/1, Bus Creator/1, bar_x_i/1
  Bus Creator1/1 -> States_virtual/1
  Controller/1(u_i) -> Saturation/1
  Saturation/1 -> bar_u_i/1, Bus Creator/3, bar_v/1
  Information subtracting/2(delta_vi) -> Controller/2(delta_vi)
  Information subtracting/3(s_i) -> Controller/3(s_i), Virtual sliding variable/1

== system Multi_drones_deri_compare/Controller 2/Quadcopter model ==
  u_i : Inport
  w_hat_p : Inport  Port=2
  w_hat_a : Inport  Port=3
  Add : Sum  Inputs=+-
  Add1 : Sum  Inputs=+-
  Bus Creator : BusCreator  Inputs=2
  Clock : Clock
  Quadcopter dynamics : MATLAB Function  TreatAsAtomicUnit=on
  f_a : Scope
  f_p : Scope
  quad_v : Scope
  quad_x : Scope
  v_int : Integrator  InitialCondition=[0;0;0;0;0;0]
  w_tilde_a_2 : Scope
  w_tilde_p_2 : Scope
  x_int : Integrator  InitialCondition=InitialCondition
  states_i : Outport
  wires:
  u_i/1 -> Quadcopter dynamics/2(u_i)
  Quadcopter dynamics/1(x_ddot) -> v_int/1
  x_int/1 -> Quadcopter dynamics/1(x_i), quad_x/1, Bus Creator/1
  v_int/1 -> Bus Creator/2, quad_v/1, Quadcopter dynamics/4(v_i), x_int/1
  Bus Creator/1 -> states_i/1
  Quadcopter dynamics/2(w_a) -> Add/1, f_a/1
  w_hat_a/1 -> Add/2
  Add/1 -> w_tilde_a_2/1
  Clock/1 -> Quadcopter dynamics/3(t)
  Quadcopter dynamics/3(w_p) -> f_p/1, Add1/1
  w_hat_p/1 -> Add1/2
  Add1/1 -> w_tilde_p_2/1

== system Multi_drones_deri_compare/Controller 3/Controller ==
  note: Change the serial number here
  note: Change the serial number here
  note: Change the serial number here
  states_i : Inport
  ref_x_p : Inport  Port=2
  psi_id : Inport  Port=3
  Attitude controller : Subsystem
      settings: PortSchema="{\"entries\":[{\"content\":{\"sides\":[{\"content\":{\"connectorIds\":[\"In1\",\"In2\",\"In3\"]},\"type\":\"ConnectorPlacement.EquallySpacedRectSide\",\"uuid\":\"fa62b1eb-ed3d-4a84-b897-b51f17bb9d42\"},{\"content\":{\"connectorIds\":[\"Out1\"],\"side\":\"RIGHT\"},\"type\":\"ConnectorPlacement.EquallySpacedRectSide\",\"uuid\":\"9b6b7a3c-e484-45bf-bd32-fe40ffeb0d28\"},{\"content\":{\"connectorIds\":[\"Out2\"],\"side\":\"TOP\"},\"type\":\"ConnectorPlacement.EquallySpacedRectSide\",\"uuid\":\"d1ffdbb9-18c9-4f2c-95a6-bf4c2ab27347\"}]},\"type\":\"ConnectorPlacement.EquallySpacedConnector\",\"uuid\":\"2804a1df-60db-43d6-95d2-4687dde4bd06\"}],\"packageUris\":[\"http://schema.mathworks.com/mf0/Connector/R2020b\"],\"version\":\"1.0\"}"
  Constant : Constant  Value=13.72  VectorParams1D=off
  Manual Switch : ManualSwitch
  Nominal control calculation : MATLAB Function  TreatAsAtomicUnit=on
  Position controller1 : Subsystem
      settings: PortSchema="{\"entries\":[{\"content\":{\"sides\":[{\"content\":{\"connectorIds\":[\"In1\",\"In2\",\"In3\"]},\"type\":\"ConnectorPlacement.EquallySpacedRectSide\",\"uuid\":\"6f6db54a-065c-4c68-96d3-ce6f9528f7c2\"},{\"content\":{\"connectorIds\":[\"Out1\"],\"side\":\"RIGHT\"},\"type\":\"ConnectorPlacement.EquallySpacedRectSide\",\"uuid\":\"eab021de-0481-49e0-8239-dbc5993eb5fa\"},{\"content\":{\"connectorIds\":[\"Out2\"],\"side\":\"TOP\"},\"type\":\"ConnectorPlacement.EquallySpacedRectSide\",\"uuid\":\"c7d044cf-1b8b-40e5-8601-940ebebd0ccb\"},{\"content\":{\"connectorIds\":[],\"side\":\"BOTTOM\"},\"type\":\"ConnectorPlacement.EquallySpacedRectSide\",\"uuid\":\"6c5daa93-b438-4c34-9741-3ab1f6346320\"}]},\"type\":\"ConnectorPlacement.EquallySpacedConnector\",\"uuid\":\"bb7db914-9823-41d6-a8ba-39b4d2976335\"}],\"packageUris\":[\"http://schema.mathworks.com/mf0/Connector/R2020b\"],\"version\":\"1.0\"}"
  Real control input : MATLAB Function  TreatAsAtomicUnit=on
  Reverse calculation : Subsystem
      settings: PortSchema="{\"entries\":[{\"content\":{\"sides\":[{\"content\":{\"connectorIds\":[\"In1\",\"In2\"]},\"type\":\"ConnectorPlacement.EquallySpacedRectSide\",\"uuid\":\"a324fb00-881d-40c1-b7da-a9c7871d46ce\"},{\"content\":{\"connectorIds\":[\"Out1\",\"Out2\"],\"side\":\"RIGHT\"},\"type\":\"ConnectorPlacement.EquallySpacedRectSide\",\"uuid\":\"58739d0b-b2b3-44e8-8796-6553ce8d5a15\"},{\"content\":{\"connectorIds\":[\"In3\"],\"side\":\"TOP\"},\"type\":\"ConnectorPlacement.EquallySpacedRectSide\",\"uuid\":\"8c9acd48-a842-4889-b739-8799f04ac800\"}]},\"type\":\"ConnectorPlacement.EquallySpacedConnector\",\"uuid\":\"9c847f57-6425-42e5-8be7-b64809e08636\"}],\"packageUris\":[\"http://schema.mathworks.com/mf0/Connector/R2020b\"],\"version\":\"1.0\"}"
  Scope : Scope
  T_id : Scope
  atti_ref : Scope
  u : Scope
  u_ip : Scope
  u_nom_a : Scope
  u_nom_p : Scope
  u_i : Outport
  w_hat_p : Outport  Port=2
  w_hat_a : Outport  Port=3
  wires:
  Attitude controller/1(u_I_a) -> Real control input/1(u_i_a)
  ref_x_p/1 -> Position controller1/2(ref_x_p)
  states_i/1 -> Position controller1/1(states_i), Reverse calculation/3(states_i), Attitude controller/1(states_i), Nominal control calculation/1(states_i)
  Nominal control calculation/1(u_nom_p) -> Position controller1/3(u_nom_p), u_nom_p/1
  Nominal control calculation/2(u_nom_a) -> Attitude controller/3(u_nom_a), u_nom_a/1
  Position controller1/1(u_i_p) -> Reverse calculation/2(u_ip), u_ip/1
  Reverse calculation/1(atti_ref) -> Attitude controller/2(atti_ref), atti_ref/1
  Position controller1/2(w_hat_p) -> w_hat_p/1
  Attitude controller/2(w_hat_a) -> w_hat_a/1
  Constant/1 -> Manual Switch/2
  Reverse calculation/2(T_i_d) -> Manual Switch/1
  Manual Switch/1 -> T_id/1, Real control input/2(T_id)
  Real control input/2(u_i) -> Nominal control calculation/2(u_i), u/1, u_i/1
  Real control input/1(tau_i) -> Scope/1
  psi_id/1 -> Reverse calculation/1(psi_id)

== system Multi_drones_deri_compare/Controller 3/High-level system ==
  L : Inport
  info_commu : Inport  Port=2
  bar_delta : Inport  Port=3
  a_d : Inport  Port=4
  Bus Creator : BusCreator  Inputs=3
  Bus Creator1 : BusCreator  Inputs=2
  Controller : MATLAB Function  TreatAsAtomicUnit=on
  Information subtracting : MATLAB Function  TreatAsAtomicUnit=on
  Saturation : Saturate  UpperLimit=0.2  LowerLimit=-0.2
  Virtual sliding variable : Scope
  Virtual tracking error : Scope
  bar_u_i : Scope
  bar_v : Integrator  InitialCondition=[0;0;0]  ContinuousStateAttributes='speed'
  bar_v_i : Scope
  bar_x : Integrator  Tag=Position_x1  InitialCondition=InitialCondition  ContinuousStateAttributes='position'
  bar_x_i : Scope
  new_ref : Outport
  States_virtual : Outport  Port=2
  wires:
  Information subtracting/1(delta_xi) -> Controller/1(delta_xi), Virtual tracking error/1
  Information subtracting/4(sat_dot) -> Controller/4(sat_dot)
  info_commu/1 -> Information subtracting/2(info_commu)
  bar_delta/1 -> Information subtracting/3(bar_delta)
  L/1 -> Information subtracting/1(L)
  a_d/1 -> Controller/5(a_di)
  bar_v/1 -> Bus Creator1/2, bar_v_i/1, Bus Creator/2, bar_x/1
  Bus Creator/1 -> new_ref/1
  bar_x/1 -> Bus Creator1/1, Bus Creator/1, bar_x_i/1
  Bus Creator1/1 -> States_virtual/1
  Controller/1(u_i) -> Saturation/1
  Saturation/1 -> bar_u_i/1, Bus Creator/3, bar_v/1
  Information subtracting/2(delta_vi) -> Controller/2(delta_vi)
  Information subtracting/3(s_i) -> Controller/3(s_i), Virtual sliding variable/1

== system Multi_drones_deri_compare/Controller 3/Quadcopter model ==
  u_i : Inport
  w_hat_p : Inport  Port=2
  w_hat_a : Inport  Port=3
  Add : Sum  Inputs=+-
  Add1 : Sum  Inputs=+-
  Bus Creator : BusCreator  Inputs=2
  Clock : Clock
  Quadcopter dynamics : MATLAB Function  TreatAsAtomicUnit=on
  f_a : Scope
  f_p : Scope
  quad_v : Scope
  quad_x : Scope
  v_int : Integrator  InitialCondition=[0;0;0;0;0;0]
  w_tilde_a : Scope
  w_tilde_p : Scope
  x_int : Integrator  InitialCondition=InitialCondition
  states_i : Outport
  wires:
  u_i/1 -> Quadcopter dynamics/2(u_i)
  Quadcopter dynamics/1(x_ddot) -> v_int/1
  x_int/1 -> Quadcopter dynamics/1(x_i), quad_x/1, Bus Creator/1
  v_int/1 -> Bus Creator/2, quad_v/1, Quadcopter dynamics/4(v_i), x_int/1
  Bus Creator/1 -> states_i/1
  Quadcopter dynamics/2(w_a) -> Add/1, f_a/1
  w_hat_a/1 -> Add/2
  Add/1 -> w_tilde_a/1
  Clock/1 -> Quadcopter dynamics/3(t)
  Quadcopter dynamics/3(w_p) -> f_p/1, Add1/1
  w_hat_p/1 -> Add1/2
  Add1/1 -> w_tilde_p/1

== system Multi_drones_deri_compare/Controller 4/Controller ==
  note: Change the serial number here
  note: Change the serial number here
  note: Change the serial number here
  states_i : Inport
  ref_x_p : Inport  Port=2
  psi_id : Inport  Port=3
  Attitude controller : Subsystem
      settings: PortSchema="{\"entries\":[{\"content\":{\"sides\":[{\"content\":{\"connectorIds\":[\"In1\",\"In2\",\"In3\"]},\"type\":\"ConnectorPlacement.EquallySpacedRectSide\",\"uuid\":\"fa62b1eb-ed3d-4a84-b897-b51f17bb9d42\"},{\"content\":{\"connectorIds\":[\"Out1\"],\"side\":\"RIGHT\"},\"type\":\"ConnectorPlacement.EquallySpacedRectSide\",\"uuid\":\"9b6b7a3c-e484-45bf-bd32-fe40ffeb0d28\"},{\"content\":{\"connectorIds\":[\"Out2\"],\"side\":\"TOP\"},\"type\":\"ConnectorPlacement.EquallySpacedRectSide\",\"uuid\":\"d1ffdbb9-18c9-4f2c-95a6-bf4c2ab27347\"}]},\"type\":\"ConnectorPlacement.EquallySpacedConnector\",\"uuid\":\"2804a1df-60db-43d6-95d2-4687dde4bd06\"}],\"packageUris\":[\"http://schema.mathworks.com/mf0/Connector/R2020b\"],\"version\":\"1.0\"}"
  Constant : Constant  Value=13.72  VectorParams1D=off
  Manual Switch : ManualSwitch
  Nominal control calculation : MATLAB Function  TreatAsAtomicUnit=on
  Position controller1 : Subsystem
      settings: PortSchema="{\"entries\":[{\"content\":{\"sides\":[{\"content\":{\"connectorIds\":[\"In1\",\"In2\",\"In3\"]},\"type\":\"ConnectorPlacement.EquallySpacedRectSide\",\"uuid\":\"6f6db54a-065c-4c68-96d3-ce6f9528f7c2\"},{\"content\":{\"connectorIds\":[\"Out1\"],\"side\":\"RIGHT\"},\"type\":\"ConnectorPlacement.EquallySpacedRectSide\",\"uuid\":\"eab021de-0481-49e0-8239-dbc5993eb5fa\"},{\"content\":{\"connectorIds\":[\"Out2\"],\"side\":\"TOP\"},\"type\":\"ConnectorPlacement.EquallySpacedRectSide\",\"uuid\":\"c7d044cf-1b8b-40e5-8601-940ebebd0ccb\"},{\"content\":{\"connectorIds\":[],\"side\":\"BOTTOM\"},\"type\":\"ConnectorPlacement.EquallySpacedRectSide\",\"uuid\":\"6c5daa93-b438-4c34-9741-3ab1f6346320\"}]},\"type\":\"ConnectorPlacement.EquallySpacedConnector\",\"uuid\":\"bb7db914-9823-41d6-a8ba-39b4d2976335\"}],\"packageUris\":[\"http://schema.mathworks.com/mf0/Connector/R2020b\"],\"version\":\"1.0\"}"
  Real control input : MATLAB Function  TreatAsAtomicUnit=on
  Reverse calculation : Subsystem
      settings: PortSchema="{\"entries\":[{\"content\":{\"sides\":[{\"content\":{\"connectorIds\":[\"In1\",\"In2\"]},\"type\":\"ConnectorPlacement.EquallySpacedRectSide\",\"uuid\":\"a324fb00-881d-40c1-b7da-a9c7871d46ce\"},{\"content\":{\"connectorIds\":[\"Out1\",\"Out2\"],\"side\":\"RIGHT\"},\"type\":\"ConnectorPlacement.EquallySpacedRectSide\",\"uuid\":\"58739d0b-b2b3-44e8-8796-6553ce8d5a15\"},{\"content\":{\"connectorIds\":[\"In3\"],\"side\":\"TOP\"},\"type\":\"ConnectorPlacement.EquallySpacedRectSide\",\"uuid\":\"8c9acd48-a842-4889-b739-8799f04ac800\"}]},\"type\":\"ConnectorPlacement.EquallySpacedConnector\",\"uuid\":\"9c847f57-6425-42e5-8be7-b64809e08636\"}],\"packageUris\":[\"http://schema.mathworks.com/mf0/Connector/R2020b\"],\"version\":\"1.0\"}"
  Scope : Scope
  T_id : Scope
  atti_ref : Scope
  u : Scope
  u_ip : Scope
  u_nom_a : Scope
  u_nom_p : Scope
  u_i : Outport
  w_hat_p : Outport  Port=2
  w_hat_a : Outport  Port=3
  wires:
  Attitude controller/1(u_I_a) -> Real control input/1(u_i_a)
  ref_x_p/1 -> Position controller1/2(ref_x_p)
  states_i/1 -> Position controller1/1(states_i), Reverse calculation/3(states_i), Attitude controller/1(states_i), Nominal control calculation/1(states_i)
  Nominal control calculation/1(u_nom_p) -> Position controller1/3(u_nom_p), u_nom_p/1
  Nominal control calculation/2(u_nom_a) -> Attitude controller/3(u_nom_a), u_nom_a/1
  Position controller1/1(u_i_p) -> Reverse calculation/2(u_ip), u_ip/1
  Reverse calculation/1(atti_ref) -> Attitude controller/2(atti_ref), atti_ref/1
  Position controller1/2(w_hat_p) -> w_hat_p/1
  Attitude controller/2(w_hat_a) -> w_hat_a/1
  Constant/1 -> Manual Switch/2
  Reverse calculation/2(T_i_d) -> Manual Switch/1
  Manual Switch/1 -> T_id/1, Real control input/2(T_id)
  Real control input/2(u_i) -> Nominal control calculation/2(u_i), u/1, u_i/1
  Real control input/1(tau_i) -> Scope/1
  psi_id/1 -> Reverse calculation/1(psi_id)
